simulink model "setup_ipm_shaping"  (R2024b)
settings: Solver=FixedStepAuto  StartTime=0.0  StopTime=1300  FixedStep=1  RelTol=1e-3
values from neighbouring files (symbols this model uses):
  c_delay_golden = 1    [seq.m]
  c_waveform = 3    [seq.m]
  LSB = 1/(2^14)    (= 6.103515625e-05)    [seq.m]
libraries: simulink x6
settings Model: PauseTimes=180  Creator=usradmin  LastModifiedBy=jose.sanchez
settings OptimizationCC: BlockReduction=off  ConditionallyExecuteInputs=off  DefaultParameterBehavior=Inlined
settings DebuggingCC: AlgebraicLoopMsg=error
settings HardwareCC: ProdBitPerPointer=32  ProdBitPerSizeT=32  ProdBitPerPtrDiffT=32  ProdLargestAtomicFloat=None  ProdIntDivRoundTo=Undefined  ProdEndianess=Unspecified  ProdWordSize=32  ProdHWDeviceType=ASIC/FPGA->ASIC/FPGA  TargetBitPerLong=64  TargetBitPerPointer=64  TargetBitPerSizeT=64  TargetBitPerPtrDiffT=64  TargetLongLongMode=on  TargetIntDivRoundTo=Zero  TargetEndianess=LittleEndian  TargetWordSize=64  TargetHWDeviceType=Custom Processor->MATLAB Host Computer  ProdEqTarget=off
settings RTWCC: GPUComputeCapability=3.5

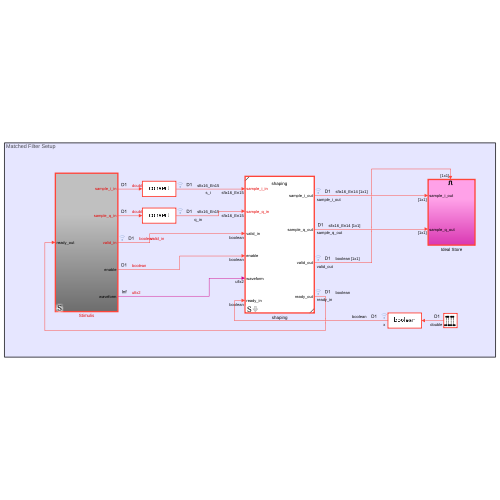
[thumbnail: Simulink's stored preview of the top-level diagram]
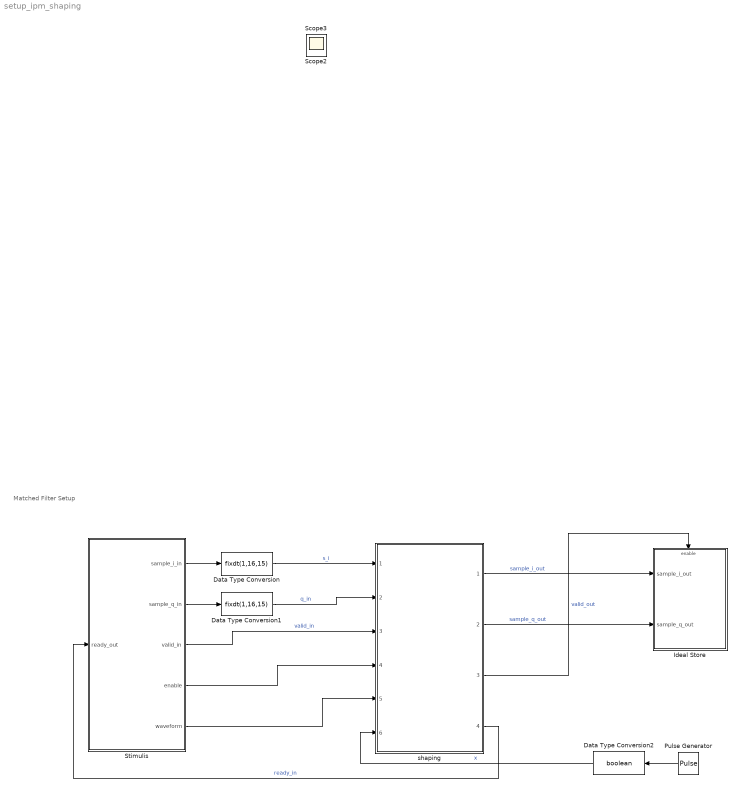
== system setup_ipm_shaping ==
  note: Matched Filter Setup
  Data Type Conversion : DataTypeConversion  OutDataTypeStr=fixdt(1,16,15)  SaturateOnIntegerOverflow=off  RndMeth=Floor
  Data Type Conversion1 : DataTypeConversion  OutDataTypeStr=fixdt(1,16,15)  SaturateOnIntegerOverflow=off  RndMeth=Floor
  Data Type Conversion2 : DataTypeConversion  OutDataTypeStr=boolean  SaturateOnIntegerOverflow=off  RndMeth=Floor
  Ideal Store : Subsystem
  Pulse Generator : DiscretePulseGenerator  Period=200  PulseWidth=100  PhaseDelay=50
  Stimulis : Subsystem
  shaping : Subsystem  ReferencedSubsystem=shaping  c_srrc_coef=c_srrc_coef  c_inter_1_coef=c_int1_coef  c_inter_2_coef=c_int2_coef
  Scope2 : Scope
  Scope3 : Scope
  wires:
  Stimulis/1(sample_i_in) -> Data Type Conversion/1
  Stimulis/2(sample_q_in) -> Data Type Conversion1/1
  Stimulis/3(valid_in) -> shaping/3  "valid_in"
  shaping/1 -> Ideal Store/1(sample_i_out)  "sample_i_out"
  shaping/2 -> Ideal Store/2(sample_q_out)  "sample_q_out"
  Data Type Conversion/1 -> shaping/1  "s_i"
  Data Type Conversion1/1 -> shaping/2  "q_in"
  shaping/4 -> Stimulis/1(ready_out)  "ready_in"
  Stimulis/4(enable) -> shaping/4
  Stimulis/5(waveform) -> shaping/5
  shaping/3 -> Ideal Store/Enable  "valid_out"
  Pulse Generator/1 -> Data Type Conversion2/1
  Data Type Conversion2/1 -> shaping/6  "x"

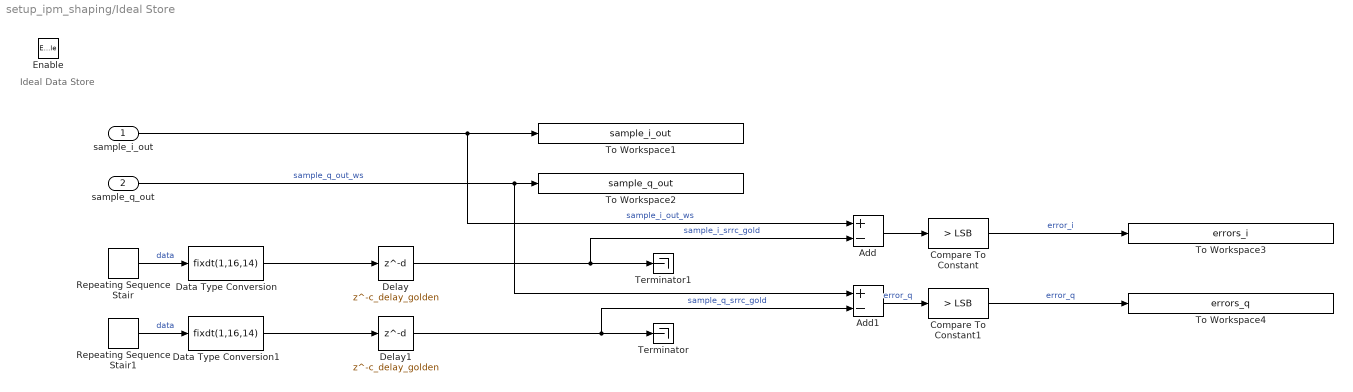
== system setup_ipm_shaping/Ideal Store ==
  note: Ideal Data Store
  sample_i_out : Inport
  sample_q_out : Inport  Port=2
  Enable : EnablePort
  Add : Sum  Inputs=+-
  Add1 : Sum  Inputs=+-
  Compare To Constant : simulink/Logic and Bit Operations/Compare To Constant  relop=>  const=LSB  OutDataTypeStr=boolean
  Compare To Constant1 : simulink/Logic and Bit Operations/Compare To Constant  relop=>  const=LSB  OutDataTypeStr=boolean
  Data Type Conversion : DataTypeConversion  OutDataTypeStr=fixdt(1,16,14)  SaturateOnIntegerOverflow=off  RndMeth=Floor
  Data Type Conversion1 : DataTypeConversion  OutDataTypeStr=fixdt(1,16,14)  SaturateOnIntegerOverflow=off  RndMeth=Floor
  Delay : Delay  DelayLength=c_delay_golden
  Delay1 : Delay  DelayLength=c_delay_golden
  Repeating Sequence Stair : simulink/Sources/Repeating Sequence Stair  OutValues=sample_i_golden  tsamp=-1  OutMin=[]  OutMax=[]  OutDataTypeStr=double  OutputDataTypeScalingMode=double  OutDataType=fixdt(0,8)  ConRadixGroup=Best Precision: Vector-wise  OutScaling=2^-12
  Repeating Sequence Stair1 : simulink/Sources/Repeating Sequence Stair  OutValues=sample_q_golden  tsamp=-1  OutMin=[]  OutMax=[]  OutDataTypeStr=double  OutputDataTypeScalingMode=double  OutDataType=fixdt(0,8)  ConRadixGroup=Best Precision: Vector-wise  OutScaling=2^-12
  Terminator : Terminator
  Terminator1 : Terminator
  To Workspace1 : ToWorkspace  VariableName=sample_i_out  SampleTime=-1
      settings: Save2DSignal=2-D array (concatenate along first dimension)
  To Workspace2 : ToWorkspace  VariableName=sample_q_out  SampleTime=-1
      settings: Save2DSignal=2-D array (concatenate along first dimension)
  To Workspace3 : ToWorkspace  VariableName=errors_i  SampleTime=-1
      settings: Save2DSignal=2-D array (concatenate along first dimension)
  To Workspace4 : ToWorkspace  VariableName=errors_q  SampleTime=-1
      settings: Save2DSignal=2-D array (concatenate along first dimension)
  wires:
  sample_i_out/1 -> Add/1, To Workspace1/1  "sample_i_out_ws"
  sample_q_out/1 -> Add1/1, To Workspace2/1  "sample_q_out_ws"
  Repeating Sequence Stair/1 -> Data Type Conversion/1  "data"
  Repeating Sequence Stair1/1 -> Data Type Conversion1/1  "data"
  Delay1/1 -> Add1/2, Terminator/1  "sample_q_srrc_gold"
  Delay/1 -> Add/2, Terminator1/1  "sample_i_srrc_gold"
  Data Type Conversion/1 -> Delay/1
  Data Type Conversion1/1 -> Delay1/1
  Add/1 -> Compare To Constant/1
  Add1/1 -> Compare To Constant1/1  "error_q"
  Compare To Constant/1 -> To Workspace3/1  "error_i"
  Compare To Constant1/1 -> To Workspace4/1  "error_q"

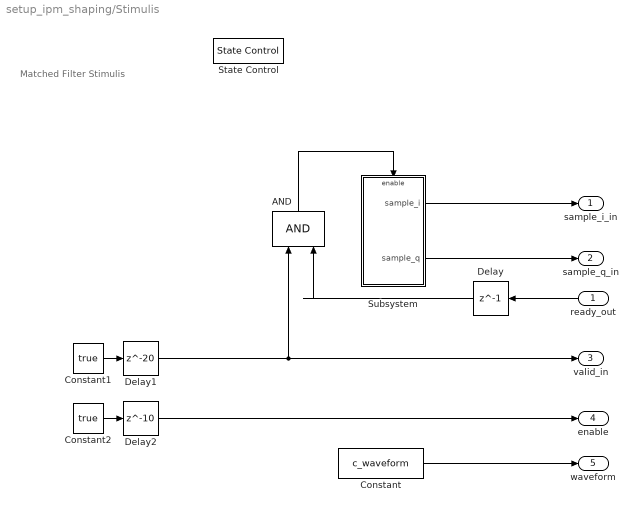
== system setup_ipm_shaping/Stimulis ==
  note: Matched Filter Stimulis
  ready_out : Inport
  AND : Logic  IconShape=distinctive  AllPortsSameDT=off  OutDataTypeStr=boolean
  Constant : Constant  Value=c_waveform  OutDataTypeStr=fixdt(0,2,0)
  Constant1 : Constant  Value=true  OutDataTypeStr=boolean
  Constant2 : Constant  Value=true  OutDataTypeStr=boolean
  Delay : Delay  DelayLength=1
  Delay1 : Delay  DelayLength=20
  Delay2 : Delay  DelayLength=10
  State Control : StateControl  StateControl=Synchronous
  Subsystem : Subsystem
  sample_i_in : Outport  VectorParamsAs1DForOutWhenUnconnected=off
  sample_q_in : Outport  Port=2  VectorParamsAs1DForOutWhenUnconnected=off
  valid_in : Outport  Port=3  VectorParamsAs1DForOutWhenUnconnected=off
  enable : Outport  Port=4
  waveform : Outport  Port=5  OutMin=[0]  OutMax=[3]  OutDataTypeStr=fixdt(0,2)
  wires:
  Subsystem/1(sample_i) -> sample_i_in/1
  Subsystem/2(sample_q) -> sample_q_in/1
  Constant/1 -> waveform/1
  Delay2/1 -> enable/1
  ready_out/1 -> Delay/1
  AND/1 -> Subsystem/Enable
  Delay1/1 -> AND/1, valid_in/1
  Delay/1 -> AND/2
  Constant1/1 -> Delay1/1
  Constant2/1 -> Delay2/1

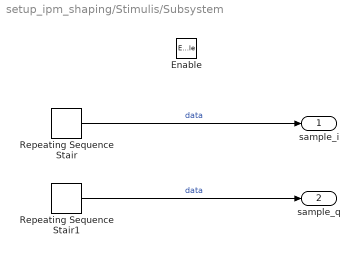
== system setup_ipm_shaping/Stimulis/Subsystem ==
  Enable : EnablePort
  Repeating Sequence Stair : simulink/Sources/Repeating Sequence Stair  OutValues=sample_i  tsamp=1  OutMin=[]  OutMax=[]  OutDataTypeStr=double  OutputDataTypeScalingMode=double  OutDataType=fixdt(0,8)  ConRadixGroup=Best Precision: Vector-wise  OutScaling=2^-12
  Repeating Sequence Stair1 : simulink/Sources/Repeating Sequence Stair  OutValues=sample_q  tsamp=1  OutMin=[]  OutMax=[]  OutDataTypeStr=double  OutputDataTypeScalingMode=double  OutDataType=fixdt(0,8)  ConRadixGroup=Best Precision: Vector-wise  OutScaling=2^-12
  sample_i : Outport  VectorParamsAs1DForOutWhenUnconnected=off
  sample_q : Outport  Port=2  VectorParamsAs1DForOutWhenUnconnected=off
  wires:
  Repeating Sequence Stair/1 -> sample_i/1  "data"
  Repeating Sequence Stair1/1 -> sample_q/1  "data"
